simulink model "parte4"  (R2024a)
settings: Solver=VariableStepAuto  StartTime=0.0  StopTime=20.0  RelTol=1e-3
undefined symbols (not defined in the file or in its folder): k_1, k_eu, tau_1, tau_2, tau_3, theta_1, theta_2, theta_3
settings Model: Creator=alexm  LastModifiedBy=alexm

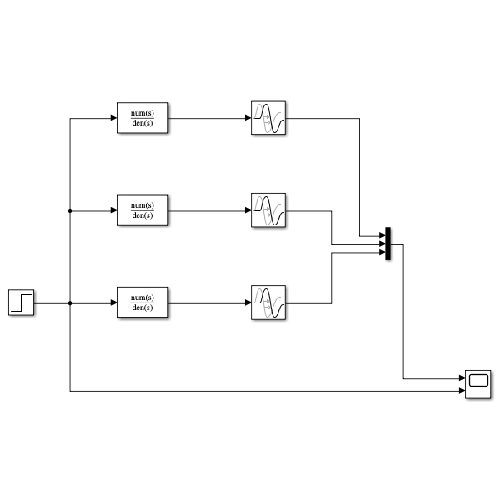
[thumbnail: Simulink's stored preview of the top-level diagram]
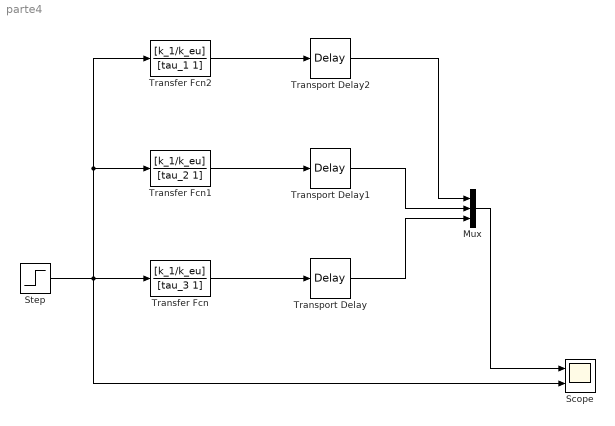
== system parte4 ==
  Mux : Mux  Inputs=3
  Scope : Scope  NumInputPorts=2
  Step : Step  After=1.5  SampleTime=0
  Transfer Fcn : TransferFcn  Numerator=[k_1/k_eu]  Denominator=[tau_3 1]
  Transfer Fcn1 : TransferFcn  Numerator=[k_1/k_eu]  Denominator=[tau_2 1]
  Transfer Fcn2 : TransferFcn  Numerator=[k_1/k_eu]  Denominator=[tau_1 1]
  Transport Delay : TransportDelay  DelayTime=[theta_3]
  Transport Delay1 : TransportDelay  DelayTime=[theta_2]
  Transport Delay2 : TransportDelay  DelayTime=[theta_1]
  wires:
  Transfer Fcn/1 -> Transport Delay/1
  Transfer Fcn1/1 -> Transport Delay1/1
  Mux/1 -> Scope/1
  Transfer Fcn2/1 -> Transport Delay2/1
  Step/1 -> Transfer Fcn2/1, Transfer Fcn1/1, Scope/2, Transfer Fcn/1
  Transport Delay/1 -> Mux/3
  Transport Delay1/1 -> Mux/2
  Transport Delay2/1 -> Mux/1
